simulink model "WC_v1"  (R2023b)
settings: Solver=FixedStepAuto  StartTime=0.0  StopTime=simtime  FixedStep=timestep  RelTol=1e-3
InitFcn:
  | % parameters= load("0 - Model\parameters2.mat");
  | %
  | % global parameters.g
  | 
  | % global g
  | %
  | % % geometry parameters
  | % global wb b a h
undefined symbols (not defined in the file or in its folder): e0, Ki, Ko, Ks, r, timestep, u0, w0, x0, xinitial, y0
libraries: simulink x9
settings Model: SimulationMode=accelerator  Creator=rober  LastModifiedBy=gianl

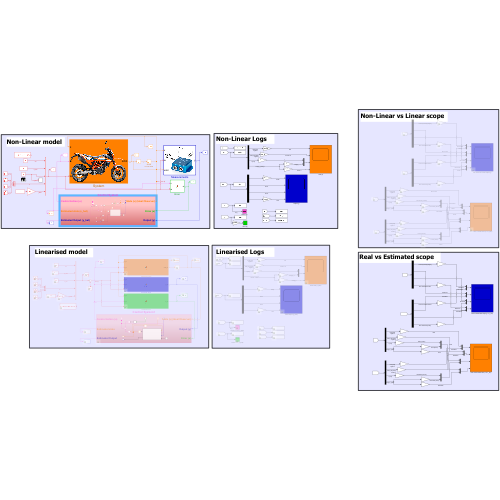
[thumbnail: Simulink's stored preview of the top-level diagram]
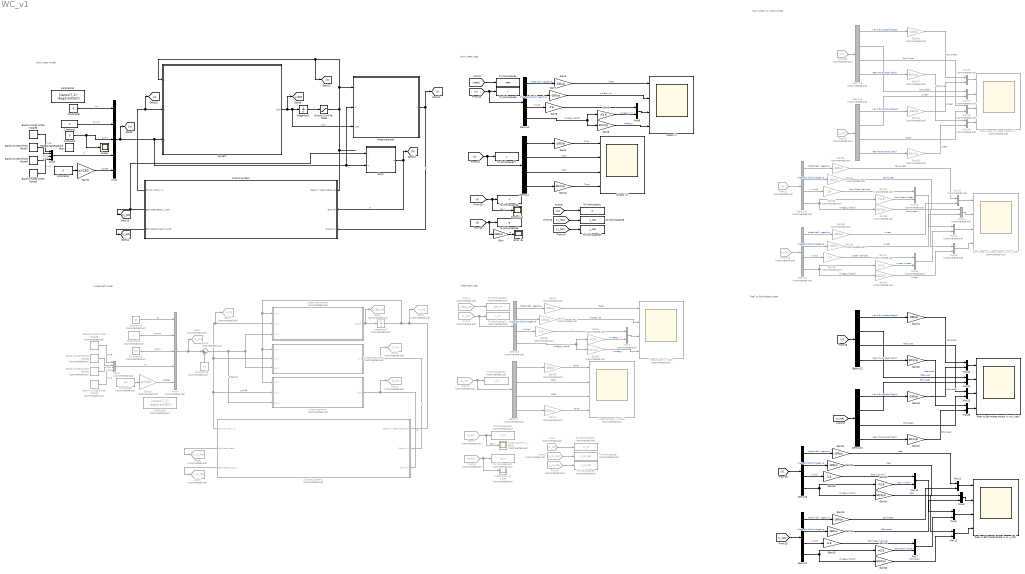
== system WC_v1 ==
  note: Linearised model
  note: Non-Linear model
  note: Non-Linear Logs
  note: Linearised Logs
  note: Real vs Estimated scope
  note: Non-Linear vs Linear scope
  Band-Limited White Noise1 : simulink/Sources/Band-Limited White Noise  Commented=on  Cov=[0.02]^2  Ts=timestep  seed=[67890]
  Band-Limited White Noise2 : simulink/Sources/Band-Limited White Noise  Commented=on  Cov=0.04*[0.01]^2  Ts=timestep  seed=[24680]
  Band-Limited White Noise3 : simulink/Sources/Band-Limited White Noise  Commented=on  Cov=[0.002]^2  Ts=timestep  seed=[23341]
  Band-Limited White Noise4 : simulink/Sources/Band-Limited White Noise  Cov=[0.02]^2  Ts=timestep  seed=[67890]
  Band-Limited White Noise5 : simulink/Sources/Band-Limited White Noise  Cov=0.04*[0.01]^2  Ts=timestep  seed=[24680]
  Band-Limited White Noise6 : simulink/Sources/Band-Limited White Noise  Cov=[0.002]^2  Ts=timestep  seed=[23341]
  Band-Limited White Noise7 : simulink/Sources/Band-Limited White Noise  Cov=[0.02]^2  Ts=timestep  seed=[13579]
  Band-Limited White Noise8 : simulink/Sources/Band-Limited White Noise  Commented=on  Cov=[0.02]^2  Ts=timestep  seed=[13579]
  Constant{1..2,8..9} (4 alike) : Constant  Value=0
  Constant10 : Constant  Value=[zeros(7,1); -deg2rad(55)]
  Constant12 : Constant  Commented=on  Value=0
  Constant13 : Constant  Commented=on  Value=-0.2
  Constant14 : Constant  Commented=on  Value=10
  Constant15 : Constant  Commented=on  Value=w0
  Constant16 : Constant  Commented=on  Value=55
  Constant3 : Constant  Commented=on  Value=[zeros(7,1); -deg2rad(55)]
  Control (u) : Scope
  Control System : Subsystem
  Control System1 : Subsystem  Commented=on
  Demux{1..2,4..5,10..11} (6 alike) : Demux
  Demux{3,6..9,12} (6 alike) : Demux  Commented=on
  Error : MATLAB Function  TreatAsAtomicUnit=on
  Error (e) : Scope
  From : From  Commented=on  GotoTag=w_lin
  From1 : From  Commented=on  GotoTag=xdot_lin
  From2 : From  Commented=on  GotoTag=x_lin
  From20 : From  Commented=on  GotoTag=y
  From21 : From  Commented=on  GotoTag=y_lin
  From22 : From  Commented=on  GotoTag=x
  From23 : From  Commented=on  GotoTag=x_lin
  From3 : From  Commented=on  GotoTag=y_lin
  From4 : From  Commented=on  GotoTag=e_lin
  From5 : From  Commented=on  GotoTag=x_lin_hat
  From6 : From  Commented=on  GotoTag=y_lin_hat
  From7 : From  Commented=on  GotoTag=u_lin
  Gain : Gain  Gain=180/pi
  Gain1 : Gain  Commented=on  Gain=r*3.6
  Gain{9..10,16,24,40,42} (6 alike) : Gain  Gain=60/2/pi
  Gain11 : Gain  Gain=-pi/180
  Gain12 : Gain  Gain=r*3.6
  Gain{5..7,13..14,21..22,41,43} (9 alike) : Gain  Gain=-180/pi
  Gain15 : Gain  Gain=3.6
  Gain17 : Gain  Commented=on  Gain=r*3.6
  Gain{2,18..19,26..27,33..34,38,44} (9 alike) : Gain  Commented=on  Gain=-180/pi
  Gain20 : Gain  Gain=r*3.6
  Gain23 : Gain  Gain=3.6
  Gain25 : Gain  Commented=on  Gain=-pi/180
  Gain28 : Gain  Commented=on  Gain=3.6
  Gain{4,29,31,36..37,39} (6 alike) : Gain  Commented=on  Gain=60/2/pi
  Gain3 : Gain  Gain=r*3.6
  Gain30 : Gain  Commented=on  Gain=3.6
  Gain32 : Gain  Commented=on  Gain=r*3.6
  Gain35 : Gain  Commented=on  Gain=3.6
  Gain8 : Gain  Gain=3.6
  Goto : Goto  Commented=on  GotoTag=w_lin
  Goto1 : Goto  Commented=on  GotoTag=xdot_lin
  Goto2 : Goto  Commented=on  GotoTag=x_lin
  Goto3 : Goto  Commented=on  GotoTag=y_lin
  Goto4 : Goto  Commented=on  GotoTag=e_lin
  Goto5 : Goto  Commented=on  GotoTag=y_lin_hat
  Goto6 : Goto  Commented=on  GotoTag=x_lin_hat
  Goto7 : Goto  Commented=on  GotoTag=u_lin
  Ground Limit for Theta : Saturate  UpperLimit=[0;inf;inf;inf]  LowerLimit=[-inf;-inf;-inf;-inf]
  Integrator2 : Integrator  InitialCondition=xinitial  UpperSaturationLimit=5  LowerSaturationLimit=-45
  Integrator3 : Integrator  Commented=on  InitialCondition=xinitial - x0  UpperSaturationLimit=5  LowerSaturationLimit=-45
  Linear Control (u_tilde) : Scope  Commented=on
  Linear Error (e_tilde) : Scope  Commented=on
  Linear Output (y_tilde) : Scope  Commented=on  NumInputPorts=4
  Linearised error : MATLAB Function  Commented=on  TreatAsAtomicUnit=on
  Linearised output : MATLAB Function  Commented=on  TreatAsAtomicUnit=on
  Linearized system : MATLAB Function  Commented=on  TreatAsAtomicUnit=on
  Measurements : MATLAB Function  TreatAsAtomicUnit=on
  Mux{1,13..22} (11 alike) : Mux  Commented=on  Inputs=2
  Mux{6..12,23..26} (11 alike) : Mux  Inputs=2
  Mux2 : Mux  Inputs=5
  Mux3 : Mux
  Mux4 : Mux  Commented=on  Inputs=5
  Mux5 : Mux  Commented=on
  Non-Linear vs Linear Output (y) : Scope  Commented=on  NumInputPorts=4
  Non-Linear vs Linear state (x vs x_tilde) : Scope  Commented=on  NumInputPorts=4
  Output (y) : Scope  NumInputPorts=4
  Real vs Estimated output (y vs y_hat) : Scope  NumInputPorts=4
  Real vs Estimated state (x vs x_hat) : Scope  NumInputPorts=4
  Repeating Sequence Stair : simulink/Sources/Repeating Sequence Stair  OutValues=[0 -0.55 0 0 0 0 0 0 0 0 -1.05 -1.05 -1.05 -1.05 0 0 0 0 0 0].'  tsamp=.5  OutMin=[]  OutMax=[]  OutDataTypeStr=double  OutputDataTypeScalingMode=double  OutDataType=fixdt(0,8)  ConRadixGroup=Best Precision: Vector-wise  OutScaling=2^-12
  Scope : Scope
  Sum5 : Sum  Commented=on  Inputs=|+-
  System : MATLAB Function  TreatAsAtomicUnit=on
  To Workspace1 : ToWorkspace  VariableName=w  SaveFormat=Timeseries  SampleTime=-1
  To Workspace10 : ToWorkspace  Commented=on  VariableName=w_lin  SaveFormat=Timeseries  SampleTime=-1
  To Workspace11 : ToWorkspace  Commented=on  VariableName=x_lin  SaveFormat=Timeseries  SampleTime=-1
  To Workspace12 : ToWorkspace  Commented=on  VariableName=xdot_lin  SaveFormat=Timeseries  SampleTime=-1
  To Workspace13 : ToWorkspace  Commented=on  VariableName=e_lin  SaveFormat=Timeseries  SampleTime=-1
  To Workspace14 : ToWorkspace  Commented=on  VariableName=y_lin  SaveFormat=Timeseries  SampleTime=-1
  To Workspace15 : ToWorkspace  Commented=on  VariableName=u_lin  SaveFormat=Timeseries  SampleTime=-1
  To Workspace16 : ToWorkspace  VariableName=e  SaveFormat=Timeseries  SampleTime=-1
  To Workspace17 : ToWorkspace  VariableName=y  SaveFormat=Timeseries  SampleTime=-1
  To Workspace18 : ToWorkspace  VariableName=u  SaveFormat=Timeseries  SampleTime=-1
  To Workspace19 : ToWorkspace  VariableName=x_hat  SaveFormat=Timeseries  SampleTime=-1
  To Workspace20 : ToWorkspace  VariableName=y_hat  SaveFormat=Timeseries  SampleTime=-1
  To Workspace3 : ToWorkspace  VariableName=x  SaveFormat=Timeseries  SampleTime=-1
  To Workspace4 : ToWorkspace  VariableName=xdot  SaveFormat=Timeseries  SampleTime=-1
  To Workspace8 : ToWorkspace  Commented=on  VariableName=x_lin_hat  SaveFormat=Timeseries  SampleTime=-1
  To Workspace9 : ToWorkspace  Commented=on  VariableName=y_lin_hat  SaveFormat=Timeseries  SampleTime=-1
  linear state (x_tilde) : Scope  Commented=on  NumInputPorts=4
  state (x) : Scope  NumInputPorts=4
  wires:
  Constant15/1 -> Sum5/2
  Error/1(e) -> [e], Control System/2(Error (e))  "e"
  Sum5/1 -> Linearised output/3(w_lin), Linearized system/3(w_lin), Linearised error/3(w_lin)  "tilde{w}"
  Integrator2/1 -> Ground Limit for Theta/1  "x"
  Mux2/1 -> [w], Measurements/2(w), Error/2(w), System/3(w)
  System/1(xdot) -> [xdot], Measurements/3(xdot), Integrator2/1  "xdot"
  Linearized system/1(xdot_lin) -> Goto1/1, Integrator3/1
  Control System/1(Control Action (u)) -> [u], System/2(u)
  Ground Limit for Theta/1 -> [x], System/1(x), Measurements/1(x), Control System/1(State (x) (Ideal Observer))
  Gain24/1 -> Mux12/1  "Real"
  Mux9/1 -> Real vs Estimated state (x vs x_hat)/3
  Gain14/1 -> Mux8/2  "Estimated"
  Gain13/1 -> Mux11/2  "Estimated"
  Demux5/2 -> Gain22/1  "theta_dot [rad/s] negative"
  Mux8/1 -> Real vs Estimated state (x vs x_hat)/2
  Gain23/1 -> Mux10/1  "Real (vehicle)"
  Mux10/1 -> Mux9/1
  Gain21/1 -> Mux11/1  "Real"
  Demux1/3 -> Gain15/1  "v [m/s]"
  Gain15/1 -> Mux7/1  "Estimated (vehicle)"
  Gain12/1 -> Mux7/2  "Estimated (wheel)"
  Demux5/1 -> Gain21/1  "theta [rad]  negative"
  Demux1/2 -> Gain14/1  "theta_dot [rad/s] negative"
  Demux1/4 -> Gain16/1, Gain12/1  "omega_r [rad/s]"
  Gain20/1 -> Mux10/2  "Real (wheel)"
  Mux7/1 -> Mux9/2
  Demux1/1 -> Gain13/1  "theta [rad]  negative"
  Mux11/1 -> Real vs Estimated state (x vs x_hat)/1
  Gain22/1 -> Mux8/1  "Real"
  Mux12/1 -> Real vs Estimated state (x vs x_hat)/4
  Demux5/3 -> Gain23/1  "v [m/s]"
  Demux5/4 -> Gain24/1, Gain20/1  "omega_r [rad/s]"
  Gain16/1 -> Mux12/2  "Estimated"
  Mux5/1 -> Mux4/4  "nu"
  Constant16/1 -> Gain25/1
  Constant12/1 -> Mux4/2  "d_num"
  Constant13/1 -> Mux4/3  "d_mu"
  Constant14/1 -> Mux4/1  "ws"
  Gain25/1 -> Mux4/5  "r_theta"
  Mux4/1 -> Goto/1, Sum5/1
  Demux7/3 -> Linear Output (y_tilde)/3  "ACCz"
  Demux3/1 -> Gain2/1  "theta [rad]  negative"
  Demux7/2 -> Linear Output (y_tilde)/2  "ACCx"
  Gain2/1 -> linear state (x_tilde)/1  "theta"
  Demux3/2 -> Gain27/1  "theta_dot [rad/s] negative"
  Gain1/1 -> Mux1/2  "omega_r * r"
  Gain4/1 -> Linear Output (y_tilde)/4  "Tone"
  Gain29/1 -> linear state (x_tilde)/4  "omega_r"
  Demux7/4 -> Gain4/1
  Demux7/1 -> Gain26/1
  Gain26/1 -> Linear Output (y_tilde)/1  "GYRy"
  Gain28/1 -> Mux1/1  "v"
  Linearised error/1(e_lin) -> Goto4/1, Control System1/3(Error (e))  "e"
  Demux3/3 -> Gain28/1  "v [m/s]"
  Mux1/1 -> linear state (x_tilde)/3
  Control System1/1(Control Action (u)) -> Linearised output/2(u_lin), Goto7/1, Linearized system/2(u_lin), Linearised error/2(u_lin)  "u_tilde"
  Demux3/4 -> Gain29/1, Gain1/1  "omega_r [rad/s]"
  Gain27/1 -> linear state (x_tilde)/2  "d theta / dt"
  Gain11/1 -> Mux2/5  "r_theta"
  Mux3/1 -> Mux2/4  "nu"
  Constant1/1 -> Mux2/2  "d_num"
  Constant2/1 -> Scope/1, Mux2/3  "d_mu"
  Constant8/1 -> Mux2/1  "ws"
  Constant9/1 -> Gain11/1
  Measurements/1(y) -> Control System/3(Output (y)), [y]  "y"
  Control System/3(Estimated Output (y_hat)) -> [y_hat]  "y"
  Gain40/1 -> Mux26/1  "Measured"
  Mux24/1 -> Real vs Estimated output (y vs y_hat)/2
  Mux26/1 -> Real vs Estimated output (y vs y_hat)/4
  Demux11/1 -> Gain41/1  "Y-axis Gyroscope [deg/s]"
  Demux11/2 -> Mux24/1  "Measured"
  Demux11/4 -> Gain40/1  "Rear Tonewheel [rad/s]"
  Demux10/2 -> Mux24/2  "Estimated"
  Mux25/1 -> Real vs Estimated output (y vs y_hat)/3
  Demux10/4 -> Gain42/1  "Rear Tonewheel [rad/s]"
  Mux23/1 -> Real vs Estimated output (y vs y_hat)/1
  Demux11/3 -> Mux25/1  "Measured"
  Gain43/1 -> Mux23/2  "Estimated"
  Gain41/1 -> Mux23/1  "Measured"
  Gain42/1 -> Mux26/2  "Estimated"
  Demux10/1 -> Gain43/1  "Y-axis Gyroscope [deg/s]"
  Demux10/3 -> Mux25/2  "Estimated"
  Integrator3/1 -> Goto2/1, Control System1/1(State (x) (Ideal Observer)), Linearised error/1(x_lin), Linearised output/1(x_lin), Linearized system/1(x_lin)
  Linearised output/1(y_lin) -> Goto3/1, Control System1/2(Output (y))  "y"
  Control System1/2(Estimated state) -> Goto6/1
  Control System1/3(Estimated Output) -> Goto5/1
  From/1 -> To Workspace10/1
  From6/1 -> To Workspace9/1
  From5/1 -> To Workspace8/1
  From4/1 -> Linear Error (e_tilde)/1, To Workspace13/1
  From3/1 -> Demux7/1, To Workspace14/1
  From2/1 -> Demux3/1, To Workspace11/1
  From1/1 -> To Workspace12/1
  From7/1 -> Linear Control (u_tilde)/1, To Workspace15/1  "tau_r"
  [u] -> Control (u)/1, To Workspace18/1  "tau_r"
  [e] -> Gain/1, To Workspace16/1
  [x] -> Demux2/1, To Workspace3/1
  Demux2/4 -> Gain9/1, Gain3/1  "omega_r [rad/s]"
  Demux4/4 -> Gain10/1
  Gain7/1 -> state (x)/2  "d theta / dt"
  Gain8/1 -> Mux6/1  "v"
  Gain6/1 -> Output (y)/1  "GYRy"
  Gain10/1 -> Output (y)/4  "Tone"
  [xdot] -> To Workspace4/1
  Demux2/3 -> Gain8/1  "v [m/s]"
  Gain5/1 -> state (x)/1  "theta"
  Gain3/1 -> Mux6/2  "omega_r * r"
  Demux4/3 -> Output (y)/3  "ACCz"
  [y] -> Demux4/1, To Workspace17/1
  Gain9/1 -> state (x)/4  "omega_r"
  Demux4/2 -> Output (y)/2  "ACCx"
  Demux4/1 -> Gain6/1
  Mux6/1 -> state (x)/3
  Demux2/1 -> Gain5/1  "theta [rad]  negative"
  [x_hat] -> To Workspace19/1
  Demux2/2 -> Gain7/1  "theta_dot [rad/s] negative"
  [w] -> To Workspace1/1
  [y_hat] -> To Workspace20/1
  [y] -> Demux11/1
  [y_hat] -> Demux10/1
  [x] -> Demux5/1
  [x_hat] -> Demux1/1
  From20/1 -> Demux9/1
  Mux18/1 -> Non-Linear vs Linear Output (y)/3
  Demux8/4 -> Gain39/1  "Rear Tonewheel [rad/s]"
  Demux9/2 -> Mux17/1  "Non-Linear"
  From23/1 -> Demux6/1
  Demux9/1 -> Gain38/1  "Y-axis Gyroscope [deg/s]"
  Demux8/2 -> Mux17/2  "Linear"
  Demux9/3 -> Mux18/1  "Non-Linear"
  Demux9/4 -> Gain37/1  "Rear Tonewheel [rad/s]"
  Mux16/1 -> Non-Linear vs Linear Output (y)/1
  Demux12/2 -> Gain34/1  "theta_dot [rad/s] negative"
  Mux15/1 -> Non-Linear vs Linear state (x vs x_tilde)/4
  Demux12/1 -> Gain33/1  "theta [rad]  negative"
  Demux12/4 -> Gain36/1, Gain32/1  "omega_r [rad/s]"
  Demux6/2 -> Gain19/1  "theta_dot [rad/s] negative"
  Mux13/1 -> Mux22/1
  Demux6/1 -> Gain18/1  "theta [rad]  negative"
  Gain35/1 -> Mux13/1  "Non-Linear (vehicle)"
  Mux14/1 -> Non-Linear vs Linear state (x vs x_tilde)/1
  Mux21/1 -> Non-Linear vs Linear state (x vs x_tilde)/2
  Gain32/1 -> Mux13/2  "Non-Linear (wheel)"
  Gain18/1 -> Mux14/2  "Linear"
  Demux6/3 -> Gain30/1  "v [m/s]"
  From21/1 -> Demux8/1
  From22/1 -> Demux12/1
  Mux20/1 -> Mux22/2
  Gain33/1 -> Mux14/1  "Non-Linear"
  Mux19/1 -> Non-Linear vs Linear Output (y)/4
  Mux22/1 -> Non-Linear vs Linear state (x vs x_tilde)/3
  Gain36/1 -> Mux15/1  "Non-Linear"
  Gain17/1 -> Mux20/2  "Linear (wheel)"
  Gain30/1 -> Mux20/1  "Linear (vehicle)"
  Demux8/1 -> Gain44/1  "Y-axis Gyroscope [deg/s]"
  Gain44/1 -> Mux16/2  "Linear"
  Gain34/1 -> Mux21/1  "Non-Linear"
  Gain39/1 -> Mux19/2  "Linear"
  Gain38/1 -> Mux16/1  "Non-Linear"
  Demux6/4 -> Gain31/1, Gain17/1  "omega_r [rad/s]"
  Gain19/1 -> Mux21/2  "Linear"
  Gain37/1 -> Mux19/1  "Non-Linear"
  Mux17/1 -> Non-Linear vs Linear Output (y)/2
  Gain31/1 -> Mux15/2  "Linear"
  Demux8/3 -> Mux18/2  "Linear"
  Demux12/3 -> Gain35/1  "v [m/s]"
  Control System/2(Estimated state (x_hat)) -> Error/1(x), [x_hat]
  Band-Limited White Noise8/1 -> Mux5/2  "nu_x"
  Band-Limited White Noise3/1 -> Mux5/1  "nu_g"
  Band-Limited White Noise2/1 -> Mux5/4  "nu_t"
  Band-Limited White Noise1/1 -> Mux5/3  "nu_z"
  Band-Limited White Noise7/1 -> Mux3/2  "nu_x"
  Band-Limited White Noise4/1 -> Mux3/3  "nu_z"
  Band-Limited White Noise5/1 -> Mux3/4  "nu_t"
  Band-Limited White Noise6/1 -> Mux3/1  "nu_g"
  Gain/1 -> Error (e)/1  "e"

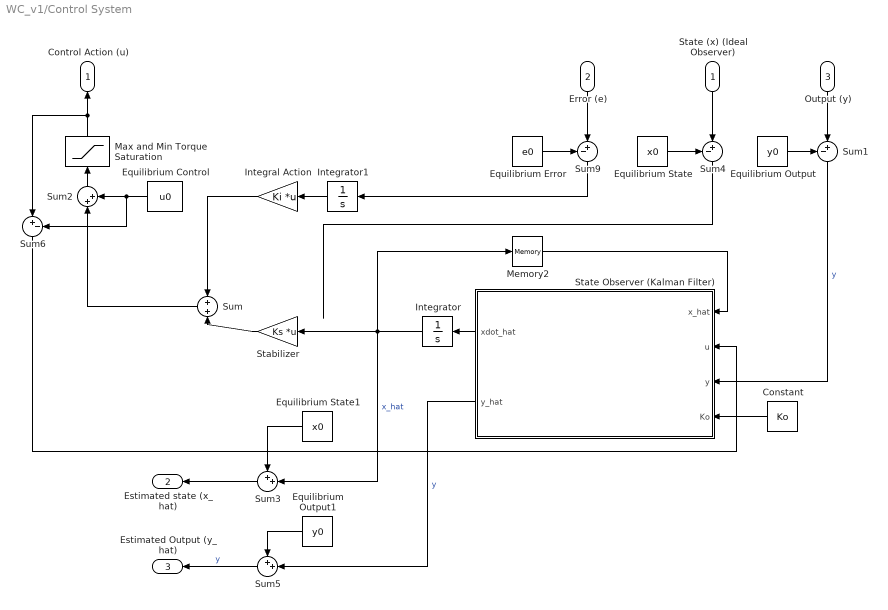
== system WC_v1/Control System ==
  State (x) (Ideal Observer) : Inport
  Error (e) : Inport  Port=2
  Output (y) : Inport  Port=3
  Constant : Constant  Value=Ko
  Equilibrium Control : Constant  Value=u0
  Equilibrium Error : Constant  Value=e0
  Equilibrium Output : Constant  Value=y0
  Equilibrium Output1 : Constant  Value=y0
  Equilibrium State : Constant  Value=x0
  Equilibrium State1 : Constant  Value=x0
  Integral Action : Gain  Gain=Ki  Multiplication=Matrix(K*u)
  Integrator : Integrator  InitialCondition=xinitial-x0
  Integrator1 : Integrator
  Max and Min Torque Saturation : Saturate  UpperLimit=754.2  LowerLimit=-200
  Memory2 : Memory  InitialCondition=xinitial-x0
  Stabilizer : Gain  Gain=Ks  Multiplication=Matrix(K*u)
  State Observer (Kalman Filter) : MATLAB Function  TreatAsAtomicUnit=on
  Sum : Sum  Inputs=+|+
  Sum1 : Sum  Inputs=-+|
  Sum2 : Sum  Inputs=|++
  Sum3 : Sum  Inputs=++|
  Sum4 : Sum  Inputs=-+|
  Sum5 : Sum  Inputs=++|
  Sum6 : Sum  Inputs=|+-
  Sum9 : Sum  Inputs=-+|
  Control Action (u) : Outport
  Estimated state (x_hat) : Outport  Port=2
  Estimated Output (y_hat) : Outport  Port=3
  wires:
  Equilibrium State/1 -> Sum4/1
  Stabilizer/1 -> Sum/2
  Equilibrium Control/1 -> Sum6/2, Sum2/2
  Sum9/1 -> Integrator1/1
  Integral Action/1 -> Sum/1
  Equilibrium Error/1 -> Sum9/1
  Error (e)/1 -> Sum9/2
  State (x) (Ideal Observer)/1 -> Sum4/2
  Sum4/1 -> ?
  Output (y)/1 -> Sum1/2
  Equilibrium Output/1 -> Sum1/1
  Equilibrium State1/1 -> Sum3/1
  Sum3/1 -> Estimated state (x_hat)/1
  Memory2/1 -> State Observer (Kalman Filter)/1(x_hat)
  Constant/1 -> State Observer (Kalman Filter)/4(Ko)
  Integrator/1 -> Sum3/2, Stabilizer/1, Memory2/1  "x_hat"
  State Observer (Kalman Filter)/1(xdot_hat) -> Integrator/1
  Sum1/1 -> State Observer (Kalman Filter)/3(y)  "y"
  Sum5/1 -> Estimated Output (y_hat)/1  "y"
  State Observer (Kalman Filter)/2(y_hat) -> Sum5/2  "y"
  Equilibrium Output1/1 -> Sum5/1
  Integrator1/1 -> Integral Action/1
  Sum/1 -> Sum2/1
  Sum2/1 -> Max and Min Torque Saturation/1
  Sum6/1 -> State Observer (Kalman Filter)/2(u)
  Max and Min Torque Saturation/1 -> Sum6/1, Control Action (u)/1

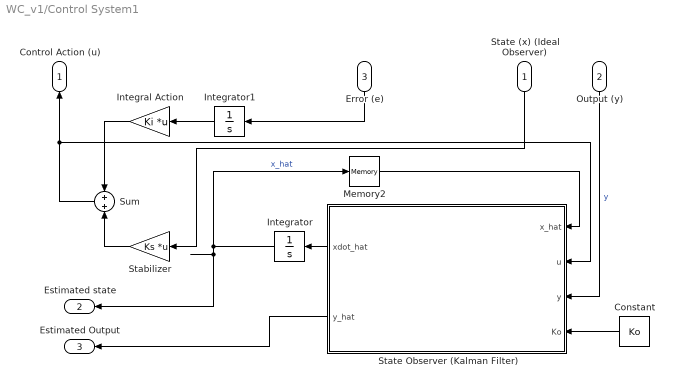
== system WC_v1/Control System1 ==
  State (x) (Ideal Observer) : Inport
  Output (y) : Inport  Port=2
  Error (e) : Inport  Port=3
  Constant : Constant  Value=Ko
  Integral Action : Gain  Gain=Ki  Multiplication=Matrix(K*u)
  Integrator : Integrator  InitialCondition=xinitial-x0
  Integrator1 : Integrator
  Memory2 : Memory  InitialCondition=xinitial-x0
  Stabilizer : Gain  Gain=Ks  Multiplication=Matrix(K*u)
  State Observer (Kalman Filter) : MATLAB Function  TreatAsAtomicUnit=on
  Sum : Sum  Inputs=+|+
  Control Action (u) : Outport
  Estimated state : Outport  Port=2
  Estimated Output : Outport  Port=3
  wires:
  Output (y)/1 -> State Observer (Kalman Filter)/3(y)  "y"
  State Observer (Kalman Filter)/2(y_hat) -> Estimated Output/1
  State (x) (Ideal Observer)/1 -> Stabilizer/1
  Sum/1 -> State Observer (Kalman Filter)/2(u), Control Action (u)/1
  Integral Action/1 -> Sum/1
  Error (e)/1 -> Integrator1/1
  Stabilizer/1 -> Sum/2
  State Observer (Kalman Filter)/1(xdot_hat) -> Integrator/1
  Integrator/1 -> Memory2/1, Estimated state/1  "x_hat"
  Memory2/1 -> State Observer (Kalman Filter)/1(x_hat)
  Constant/1 -> State Observer (Kalman Filter)/4(Ko)
  Integrator1/1 -> Integral Action/1

== matlab function WC_v1/Control System1/State Observer (Kalman Filter) ==
  data: x_hat input; xdot_hat output; u input; y input; Ko input; y_hat output
function [xdot_hat, y_hat] = Observer(x_hat,u,y,Ko)

    %% Parameters
    persistent parameters
    if isempty(parameters)
        parameters=load("0 - Model\parameters3.mat");
    end

    % Linearization matrices
    A = parameters.A;
    B1 = parameters.B1;
    B2 = parameters.B2;
    C = parameters.C;
    D1 = parameters.D1;
    D2 = parameters.D2;

    %% Exogenous Estimation
    w_hat= zeros(size(B2,2) , 1); % not estimated

    %% State Estimation

    % Estimated output
    y_hat = C*x_hat + D1*u + D2*w_hat;

    % Measurement error
    ey = y_hat - y;
    
    % Estimated dynamics
    xdot_hat = A*x_hat + B1*u + B2*w_hat - Ko*ey;

end

== matlab function WC_v1/Control System/State Observer (Kalman Filter) ==
  data: x_hat input; xdot_hat output; u input; y input; Ko input; y_hat output
function [xdot_hat, y_hat] = Observer(x_hat,u,y,Ko)

    %% Parameters
    persistent parameters
    if isempty(parameters)
        parameters=load("0 - Model\parameters3.mat");
    end

    % Linearization matrices
    A = parameters.A;
    B1 = parameters.B1;
    B2 = parameters.B2;
    C = parameters.C;
    D1 = parameters.D1;
    D2 = parameters.D2;

    %% Exogenous Estimation
    w_hat= zeros(size(B2,2) , 1); % not estimated

    %% State Estimation
    % Estimated output
    y_hat = C*x_hat + D1*u + D2*w_hat;

    %y_hat(3)=-y_hat(3);

    % Measurement error
    ey = y_hat - y;
    
    % Estimated dynamics
    xdot_hat = A*x_hat + B1*u + B2*w_hat - Ko*ey;

end

== matlab function WC_v1/Linearised output ==
  data: x_lin input; y_lin output; u_lin input; w_lin input
function y_lin = h_lin(x_lin, u_lin, w_lin)
    %% Parameters
    persistent parameters
    if isempty(parameters)
        clear parameters
        parameters=load("0 - Model\parameters3.mat");
    end
    
    % Linearization matrixes 
    C = parameters.C;
    D1 = parameters.D1;
    D2 = parameters.D2;

    %% linearized Output
    y_lin = C*x_lin + D1*u_lin + D2*w_lin;
end

== matlab function WC_v1/Linearised error ==
  data: x_lin input; e_lin output; u_lin input; w_lin input
function e_lin = he_lin(x_lin, u_lin, w_lin)

    %% Parameters
    persistent parameters
    if isempty(parameters)
        clear parameters
        parameters=load("0 - Model\parameters3.mat");
    end
    
    % Linearization matrixes 
    Ce = parameters.Ce;
    De1 = parameters.De1;
    De2 = parameters.De2;

    %% Linearized Regulated output

    e_lin = Ce*x_lin + De1*u_lin + De2*w_lin;

end

== matlab function WC_v1/System ==
  data: x input; u input; xdot output; w input
function xdot = f(x,u,w)

    %% Parameters
    persistent parameters
    if isempty(parameters)
        clear parameters
        parameters=load("0 - Model\parameters3.mat");
    end
    g= parameters.g;            %[m/s^2] gravitational acceleration

    % Motorbike geometries
    b = parameters.b;           %[m] distance between rear wheel center and COG
    a = parameters.a;           %[m] distance between front wheel center and COG
    h = parameters.h;           %[m] COG height from wheel center
    r = parameters.r;           %[m] rear wheel radius
    L = parameters.L;           %[m] bike frontal width 

    % Masses and Inertias
    mb = parameters.mb;         %[kg] bike weight + driver's weight
    mw = parameters.mw;         %[kg] wheels weight
    m = parameters.m;           %[Kg] 
    Iw = parameters.Iw;         %[Kg*m^2] wheels inertia
    I = parameters.I;           %[Kg*m^2] Total inertia at the rear wheel hub

    % Aerodynamics
    rho = parameters.rho;       %[kg/m^3] air density
    Cd = parameters.Cd;         %[-] drag coefficient

    % Pacejka coefficients
    br = parameters.br;         % stiffness factor
    cr = parameters.cr;         % shape factor 
    dr = parameters.dr;         % peak value 
    er = parameters.er;         % curvature factor
    
    %% Model
    % State
    theta = x(1);               %[rad]
    theta_d = x(2);             %[rad/s]
    v = x(3);                   %[m/s]
    omega_r = x(4);             %[rad/s]

    % Control
    tau_r = u;                  %[Nm] torque

    % Exogenous
    ws = w(1);                  %[m/s] air speed
    d_num= w(2);
    d_mu= w(3);
    
    %% Aerodynamics 
    %[m^2] cross-section
    S = (-(a+b)*sin(theta)+2*h*cos(theta))*L;       
    
    % Drag force
    D = 1/2 *rho*S*Cd*(v-ws)^2;
    
    %% Bike lengths in xy refernece
    % Center of gravity (G)
    BGx = b*cos(theta)+h*sin(theta);   %[m] CoG x coord from rear wheel hub
    BGz = h*cos(theta)-b*sin(theta);   %[m] CoG z coord from rear wheel hub

    % Front wheel center (A)
    BAx = (a+b)*cos(theta);            %[m] front wheel x coord from rear wheel hub
    BAz = -(a+b)*sin(theta);           %[m] front wheel z coord from rear wheel hub

    % Special terms that will appear frequently 
    Mx = mb*BGx + mw*BAx;
    Mz = mb*BGz + mw*BAz;
     
    %% Tyre model 

    % Slip Ratio
    lambda_r = 1 - v/(omega_r*r);    

    % Friction coefficient (Pacejka Model)
    mur = dr*sin( cr*atan( br*lambda_r - er*( br*lambda_r-atan(br*lambda_r) ) ) ) + d_mu; 
    
    %% Dynamics
    % State Evolution
    % The model has been written as LH*xdot=RH, where LH is a matrix
    % containing the terms related to xdot whereas RH is the matrix
    % containing all the constant terms and terms not related to xdot.

    LH = [1         0              0         0;
          0         1             Mz/I       0;
          0   (Mz+mur*Mx)/m        1         0;
          0   -mur*Mx*r/Iw         0         1];

    RH = [theta_d + d_num;
          1/I * (Mx*g - D*BGz - tau_r);
          1/m * (mur*(m*g-Mz*theta_d^2) - D + Mx*theta_d^2);
          1/Iw * (tau_r - mur*(m*g-Mz*theta_d^2)*r)];
    
    xdot = LH\RH;
end

== matlab function WC_v1/Measurements ==
  data: x input; y output size=4; w input; xdot input
function y = h(x,w,xdot)

    %% Parameters
    persistent parameters
    if isempty(parameters)
        clear parameters
        parameters=load("0 - Model\parameters3.mat");
    end
    g= parameters.g;        %[m/s^2] gravitational acceleration

    % Motorbike geometries
    b = parameters.b;             %[m] distance between rear wheel center and COG
    h = parameters.h;             %[m] COG height from wheel center

    %% Model

    % State
    theta = x(1);        %[rad]
    omega_r = x(4);      %[rad/s]

    % noise
    nu_g = w(4);         % noise
    nu_x = w(5);
    nu_z = w(6);
    nu_t = w(7);
    
    %% Bike lengths in xy sor
    % Center of gravity (G)
    BGx = b*cos(theta)+h*sin(theta);   %[m] x coord of COG distance from the rear wheel center
    BGz = h*cos(theta)-b*sin(theta);   %[m] y coord of COG distance from the rear wheel center
    
    %% Dynamics

    theta_d = xdot(1);
    theta_dd = xdot(2);
    v_d = xdot(3);

    %% Output
    
    y = [theta_d + nu_g ;
        v_d*cos(theta) + theta_dd*(BGz*cos(theta)+BGx*sin(theta)) - theta_d^2*(BGx*cos(theta)-BGz*sin(theta)) - g*sin(theta) + nu_x;
        v_d*sin(theta) + theta_dd*(BGz*sin(theta)-BGx*cos(theta)) - theta_d^2*(BGx*sin(theta)+BGz*cos(theta)) + g*cos(theta) + nu_z;
        omega_r*(1 + nu_t)];
end

== matlab function WC_v1/Error ==
  data: x input; w input; e output
function e = he(x,w)     
    
    theta= x(1);
    r_theta= w(8);

    e = theta - r_theta;
end

== matlab function WC_v1/Linearized system ==
  data: x_lin input; xdot_lin output; u_lin input; w_lin input
function xdot_lin = f_lin(x_lin,u_lin,w_lin)
    
    %% Parameters
    persistent parameters
    if isempty(parameters)
        clear parameters
        parameters=load("0 - Model\parameters3.mat");
    end
    
    % Linearization matrixes 
    A = parameters.A;
    B1 = parameters.B1;
    B2 = parameters.B2;

    %% Linearized State evolution
    xdot_lin = A*x_lin+B1*u_lin+B2*w_lin;
end
